simulink model "closed_loop"  (R2020b)
settings: Solver=VariableStepAuto  StartTime=0.0  StopTime=50.0  RelTol=1e-3
values from neighbouring files (symbols this model uses):
  K = 1    [lab1.m]    (also in lab1_5.m = i*1.5)
settings Model: Creator=kengoakano  LastModifiedBy=kengoakano

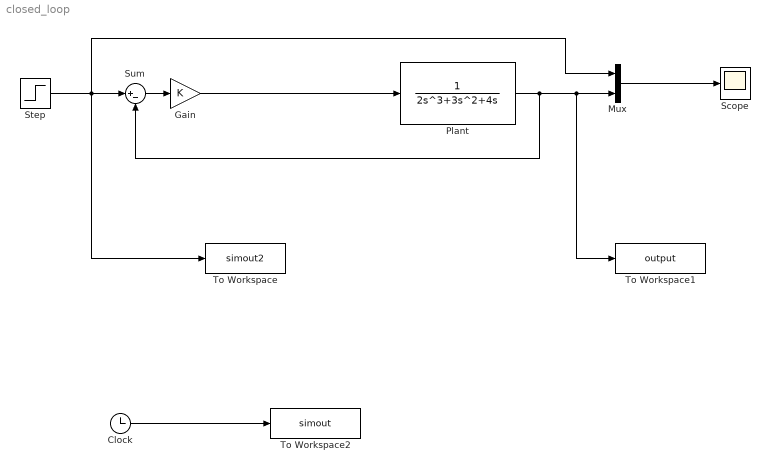
== system closed_loop ==
  Clock : Clock
  Gain : Gain  Gain=K
  Mux : Mux  Inputs=2
  Plant : TransferFcn  Denominator=[2 3 4 0]
  Scope : Scope
  Step : Step  SampleTime=0
  Sum : Sum  Inputs=|+-
  To Workspace : ToWorkspace  VariableName=simout2  SaveFormat=Timeseries  SampleTime=-1
  To Workspace1 : ToWorkspace  VariableName=output  SaveFormat=Timeseries  SampleTime=-1
  To Workspace2 : ToWorkspace  VariableName=simout  SaveFormat=Timeseries  SampleTime=-1
  wires:
  Mux/1 -> Scope/1
  Clock/1 -> To Workspace2/1
  Sum/1 -> Gain/1
  Step/1 -> To Workspace/1, Mux/1, Sum/1
  Gain/1 -> Plant/1
  Plant/1 -> To Workspace1/1, Mux/2, Sum/2
